simulink model "Act2Simulink"  (R2023b)
settings: Solver=VariableStepAuto  StartTime=0.0  StopTime=10.0  RelTol=1e-3
InitFcn:
  | ip = 0.0079; % kg*m^2
  | mc = 0.7031; % kg
  | lp = 0.3302; % m
  | mp = 0.23; % kg
  | fc = 0; % N
  | beq = 4.3; % Ns/m
  | g = 9.81; % m/s^2
  | bp = 0.0024; % Nms/rad
settings Model: Creator=adria  LastModifiedBy=adria

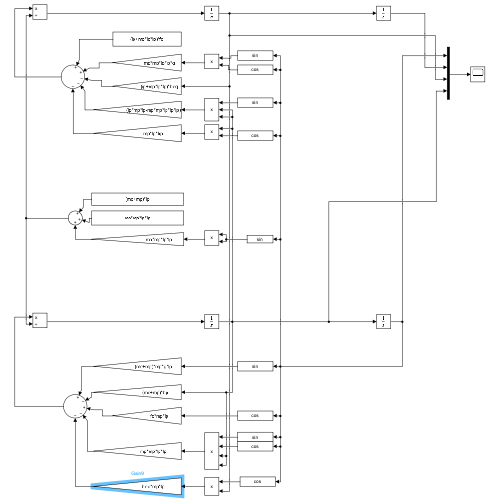
[thumbnail: Simulink's stored preview of the top-level diagram]
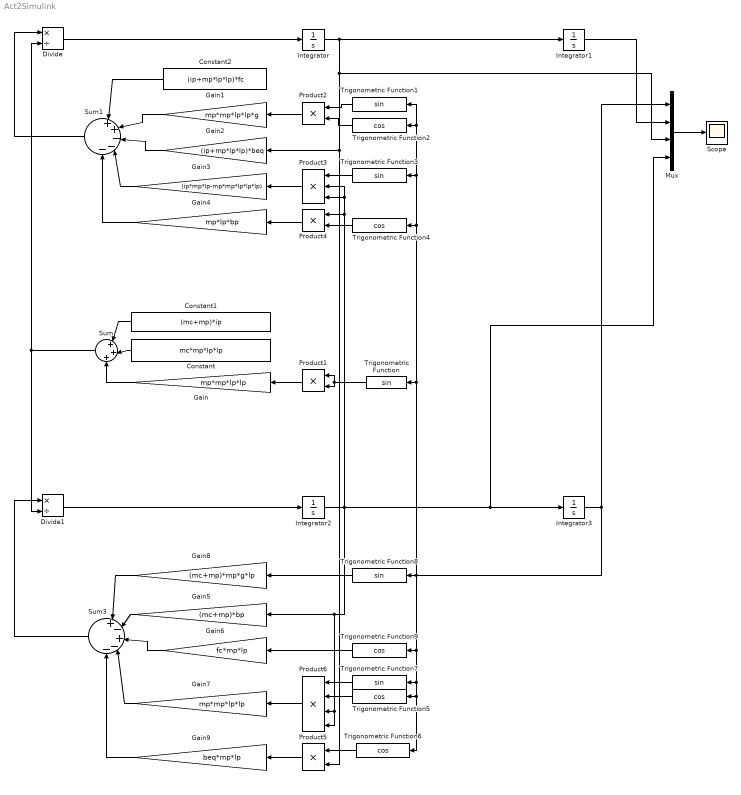
== system Act2Simulink ==
  Constant : Constant  Value=mc*mp*lp*lp
  Constant1 : Constant  Value=(mc+mp)*ip
  Constant2 : Constant  Value=(ip+mp*lp*lp)*fc
  Divide : Product  Inputs=*/
  Divide1 : Product  Inputs=*/
  Gain : Gain  Gain=mp*mp*lp*lp
  Gain1 : Gain  Gain=mp*mp*lp*lp*g
  Gain2 : Gain  Gain=(ip+mp*lp*lp)*beq
  Gain3 : Gain  Gain=(ip*mp*lp-mp*mp*lp*lp*lp)
  Gain4 : Gain  Gain=mp*lp*bp
  Gain5 : Gain  Gain=(mc+mp)*bp
  Gain6 : Gain  Gain=fc*mp*lp
  Gain7 : Gain  Gain=mp*mp*lp*lp
  Gain8 : Gain  Gain=(mc+mp)*mp*g*lp
  Gain9 : Gain  Gain=beq*mp*lp
  Integrator : Integrator
  Integrator1 : Integrator
  Integrator2 : Integrator
  Integrator3 : Integrator  InitialCondition=pi/180
  Mux : Mux
  Product{1..2,4..5} (4 alike) : Product
  Product3 : Product  Inputs=3
  Product6 : Product  Inputs=4
  Scope : Scope
  Sum : Sum  Inputs=|+|+|+
  Sum1 : Sum  Inputs=|+|+|-|-|-
  Sum3 : Sum  Inputs=|+|-|+|-|-
  Trigonometric Function{,1,3,7..8} (5 alike) : Trigonometry
  Trigonometric Function{2,4..6,9} (5 alike) : Trigonometry  Operator=cos
  wires:
  Constant1/1 -> Sum/1
  Constant/1 -> Sum/2
  Gain/1 -> Sum/3
  Trigonometric Function/1 -> Product1/2, Product1/1
  Product1/1 -> Gain/1
  Sum/1 -> Divide1/2, Divide/2
  Divide1/1 -> Integrator2/1
  Integrator2/1 -> Product6/3, Product6/4, Gain5/1, Product4/1, Product3/2, Product3/3, Mux/4, Integrator3/1
  Divide/1 -> Integrator/1
  Integrator/1 -> Mux/3, Product5/2, Gain2/1, Integrator1/1
  Sum1/1 -> Divide/1
  Constant2/1 -> Sum1/1
  Gain1/1 -> Sum1/2
  Trigonometric Function1/1 -> Product2/1
  Product2/1 -> Gain1/1
  Trigonometric Function2/1 -> Product2/2
  Gain2/1 -> Sum1/3
  Gain3/1 -> Sum1/4
  Product3/1 -> Gain3/1
  Trigonometric Function3/1 -> Product3/1
  Gain4/1 -> Sum1/5
  Product4/1 -> Gain4/1
  Trigonometric Function4/1 -> Product4/2
  Sum3/1 -> Divide1/1
  Trigonometric Function7/1 -> Product6/1
  Product6/1 -> Gain7/1
  Gain8/1 -> Sum3/1
  Trigonometric Function8/1 -> Gain8/1
  Gain5/1 -> Sum3/2
  Gain6/1 -> Sum3/3
  Trigonometric Function9/1 -> Gain6/1
  Gain7/1 -> Sum3/4
  Trigonometric Function5/1 -> Product6/2
  Product5/1 -> Gain9/1
  Trigonometric Function6/1 -> Product5/1
  Integrator3/1 -> Mux/1, Trigonometric Function6/1, Trigonometric Function5/1, Trigonometric Function7/1, Trigonometric Function9/1, Trigonometric Function8/1, Trigonometric Function1/1, Trigonometric Function2/1, Trigonometric Function3/1, Trigonometric Function4/1, Trigonometric Function/1
  Integrator1/1 -> Mux/2
  Mux/1 -> Scope/1
  Gain9/1 -> Sum3/5
